simulink model "Plant_4"  (R2024b)
settings: Solver=VariableStepAuto  StartTime=0.0  StopTime=2  RelTol=1e-3
undefined symbols (not defined in the file or in its folder): g, I1, I2, L1, L2, lc1, lc2, m1, m2
libraries: slpidlib x2, simulink x2
settings Model: Creator=Sez26  LastModifiedBy=Sez26

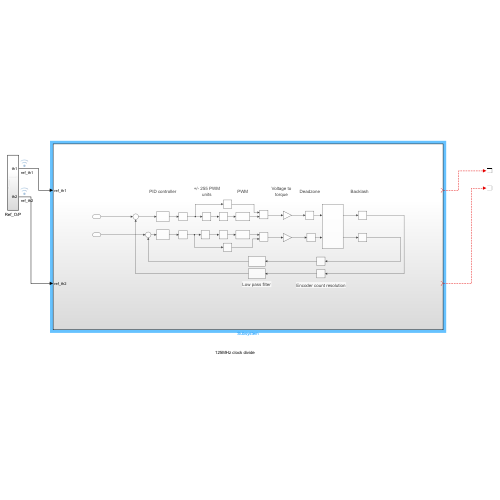
[thumbnail: Simulink's stored preview of the top-level diagram]
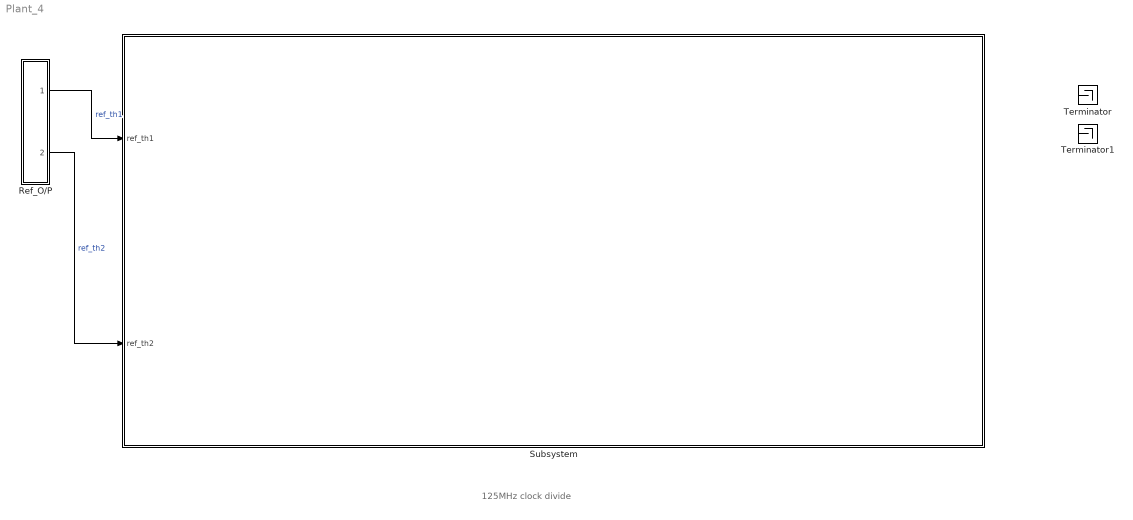
== system Plant_4 ==
  note: 125MHz clock divide
  Ref_O/P : Subsystem
  Subsystem : Subsystem
  Terminator : Terminator
  Terminator1 : Terminator
  wires:
  Ref_O/P/1(th1) -> Subsystem/1(ref_th1)  "ref_th1"
  Ref_O/P/2(th2) -> Subsystem/2(ref_th2)  "ref_th2"
  ? -> Terminator/1
  ? -> Terminator1/1

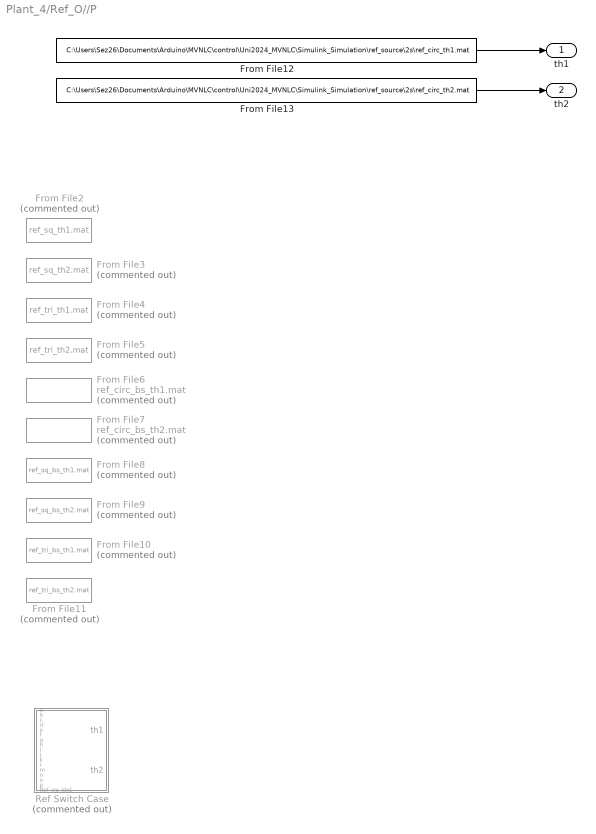
== system Plant_4/Ref_O//P ==
  From File10 : FromFile  Commented=on  FileName=ref_tri_bs_th1.mat  SampleTime=0
  From File11 : FromFile  Commented=on  FileName=ref_tri_bs_th2.mat  SampleTime=0
  From File12 : FromFile  FileName=C:\Users\Sez26\Documents\Arduino\MVNLC\control\Uni2024_MVNLC\Simulink_Simulation\ref_source\2s\ref_circ_th1.mat  SampleTime=0
  From File13 : FromFile  FileName=C:\Users\Sez26\Documents\Arduino\MVNLC\control\Uni2024_MVNLC\Simulink_Simulation\ref_source\2s\ref_circ_th2.mat  SampleTime=0
  From File2 : FromFile  Commented=on  FileName=ref_sq_th1.mat  SampleTime=0
  From File3 : FromFile  Commented=on  FileName=ref_sq_th2.mat  SampleTime=0
  From File4 : FromFile  Commented=on  FileName=ref_tri_th1.mat  SampleTime=0
  From File5 : FromFile  Commented=on  FileName=ref_tri_th2.mat  SampleTime=0
  From File6 : FromFile  Commented=on  FileName=ref_circ_bs_th1.mat  SampleTime=0
  From File7 : FromFile  Commented=on  FileName=ref_circ_bs_th2.mat  SampleTime=0
  From File8 : FromFile  Commented=on  FileName=ref_sq_bs_th1.mat  SampleTime=0
  From File9 : FromFile  Commented=on  FileName=ref_sq_bs_th2.mat  SampleTime=0
  Ref Switch Case : MATLAB Function  Commented=on  TreatAsAtomicUnit=on
  th1 : Outport
  th2 : Outport  Port=2
  wires:
  From File12/1 -> th1/1
  From File13/1 -> th2/1

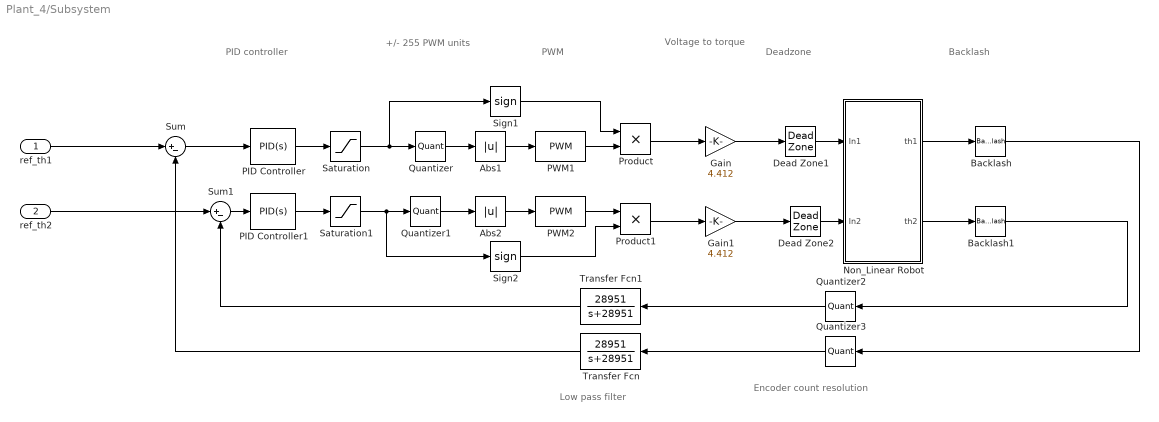
== system Plant_4/Subsystem ==
  note: PID controller
  note: +/- 255 PWM
      | units
  note: PWM
  note: Voltage to
      | torque
  note: Deadzone
  note: Low pass filter
  note: Encoder count resolution
  note: Backlash
  ref_th1 : Inport
  ref_th2 : Inport  Port=2
  Abs1 : Abs  SaturateOnIntegerOverflow=off
  Abs2 : Abs  SaturateOnIntegerOverflow=off
  Backlash : Backlash
  Backlash1 : Backlash
  Dead Zone1 : DeadZone  LowerValue=-(2.1/12)*4.4129925  UpperValue=(2.1/12)*4.4129925
  Dead Zone2 : DeadZone  LowerValue=-(2.1/12)*4.4129925  UpperValue=(2.1/12)*4.4129925
  Gain : Gain  Gain=4.412
  Gain1 : Gain  Gain=4.412
  Non_Linear Robot : Subsystem
  PID Controller : slpidlib/PID Controller  Controller=PID  Form=Parallel  TimeDomain=Continuous-time  UseExternalTs=off  SampleTime=-1  IntegratorMethod=Forward Euler  FilterMethod=Forward Euler  ControllerParametersSource=internal  P=300  I=0.1  UseKiTs=off  D=10  UseExternalDerivativeSource=off  N=100  UseFilter=on  TunerSelectOption=Transfer Function Based (PID Tuner App)  InitialConditionSource=internal  InitialConditionForIntegrator=0  InitialConditionForFilter=0  DifferentiatorICPrevScaledInput=0  ExternalReset=none  TrackingMode=off  Kt=1  LimitOutput=off  SatLimitsSource=internal  UpperSaturationLimit=1  LowerSaturationLimit=-1  LinearizeAsGain=on  AntiWindupMode=none  Kb=1  LimitIntegrator=off  UpperIntegratorSaturationLimit=inf  LowerIntegratorSaturationLimit=-inf  POutMin=[]  POutMax=[]  IOutMin=[]  IOutMax=[]  DOutMin=[]  DOutMax=[]  NOutMin=[]  NOutMax=[]  SumOutMin=[]  SumOutMax=[]  SaturationOutMin=[]  SaturationOutMax=[]  PParamMin=[]  PParamMax=[]  IParamMin=[]  IParamMax=[]  DParamMin=[]  DParamMax=[]  NParamMin=[]  NParamMax=[]  KbParamMin=[]  KbParamMax=[]  KtParamMin=[]  KtParamMax=[]  KbOutMin=[]  KbOutMax=[]  KtOutMin=[]  KtOutMax=[]  IntegratorOutMin=[]  IntegratorOutMax=[]  FilterOutMin=[]  FilterOutMax=[]  SumI1OutMin=[]  SumI1OutMax=[]  SumI2OutMin=[]  SumI2OutMax=[]  SumI3OutMin=[]  SumI3OutMax=[]  SumI4OutMin=[]  SumI4OutMax=[]  SumDOutMin=[]  SumDOutMax=[]  DifferentiatorOutMin=[]  DifferentiatorOutMax=[]  FilterDiffOutCoefMin=[]  FilterDiffOutCoefMax=[]  ReciprocalOutMin=[]  ReciprocalOutMax=[]  SumDenOutMin=[]  SumDenOutMax=[]  SumNumOutMin=[]  SumNumOutMax=[]  DivideOutMin=[]  DivideOutMax=[]  UdiffTsProdOutMin=[]  UdiffTsProdOutMax=[]  NTsProdOutMin=[]  NTsProdOutMax=[]  UintegralTsProdOutMin=[]  UintegralTsProdOutMax=[]  UngainTsProdOutMin=[]  UngainTsProdOutMax=[]  ClampingZeroOutDataTypeStr=Inherit: Inherit via back propagation  ClampingZeroOutMin=[]  ClampingZeroOutMax=[]  FilterDenConstantOutDataTypeStr=Inherit: Inherit via back propagation  FilterDenConstantOutMin=[]  FilterDenConstantOutMax=[]  PCopyOutDataTypeStr=Inherit: Inherit via back propagation  PCopyOutMin=[]  PCopyOutMax=[]  NCopyOutDataTypeStr=Inherit: Inherit via back propagation  NCopyOutMin=[]  NCopyOutMax=[]  IntegratorContinuousStateAttributes=''  IntegratorStateMustResolveToSignalObject=off  IntegratorRTWStateStorageClass=Auto  FilterContinuousStateAttributes=''  FilterStateMustResolveToSignalObject=off  FilterRTWStateStorageClass=Auto  ParallelPVariant=InternalParameters  IdealPVariant=Disabled  IVariant=InternalParameters  DVariant=InternalParameters  IntegratorVariant=Continuous  SatVariant=Disabled  AWVariant=Passthrough  PCopyVariant=Disabled  TRVariant=Disabled  FdbkBlocksVariant=Forward  IdealPFdbkVariant=Disabled  SatFdbkVariant=Disabled  DerivativeFilterVariant=ContFilter  NVariant=InternalParameters  NCopyVariant=Disabled  FilterICVariant=InternalICsFilter  IntegratorICVariant=InternalICs  ExternalResetVariant=Disabled  TRSumVariant=Passthrough  SumFdbkVariant=Disabled  SumVariant=Sum_PID  TsampFilterVariant=InternalTs  TsampNgainVariant=Passthrough  TsampIntegralVariant=Disabled_SignalSpec  ExternalSaturationOutDataTypeStr=Inherit: Same as second input  DerivativeSourceVariant=ErrorSignal  PreIntVariant=InternalPreInt
  PID Controller1 : slpidlib/PID Controller  Controller=PID  Form=Parallel  TimeDomain=Continuous-time  UseExternalTs=off  SampleTime=-1  IntegratorMethod=Forward Euler  FilterMethod=Forward Euler  ControllerParametersSource=internal  P=300  I=0.1  UseKiTs=off  D=10  UseExternalDerivativeSource=off  N=100  UseFilter=on  TunerSelectOption=Transfer Function Based (PID Tuner App)  InitialConditionSource=internal  InitialConditionForIntegrator=0  InitialConditionForFilter=0  DifferentiatorICPrevScaledInput=0  ExternalReset=none  TrackingMode=off  Kt=1  LimitOutput=off  SatLimitsSource=internal  UpperSaturationLimit=1  LowerSaturationLimit=-1  LinearizeAsGain=on  AntiWindupMode=none  Kb=1  LimitIntegrator=off  UpperIntegratorSaturationLimit=inf  LowerIntegratorSaturationLimit=-inf  POutMin=[]  POutMax=[]  IOutMin=[]  IOutMax=[]  DOutMin=[]  DOutMax=[]  NOutMin=[]  NOutMax=[]  SumOutMin=[]  SumOutMax=[]  SaturationOutMin=[]  SaturationOutMax=[]  PParamMin=[]  PParamMax=[]  IParamMin=[]  IParamMax=[]  DParamMin=[]  DParamMax=[]  NParamMin=[]  NParamMax=[]  KbParamMin=[]  KbParamMax=[]  KtParamMin=[]  KtParamMax=[]  KbOutMin=[]  KbOutMax=[]  KtOutMin=[]  KtOutMax=[]  IntegratorOutMin=[]  IntegratorOutMax=[]  FilterOutMin=[]  FilterOutMax=[]  SumI1OutMin=[]  SumI1OutMax=[]  SumI2OutMin=[]  SumI2OutMax=[]  SumI3OutMin=[]  SumI3OutMax=[]  SumI4OutMin=[]  SumI4OutMax=[]  SumDOutMin=[]  SumDOutMax=[]  DifferentiatorOutMin=[]  DifferentiatorOutMax=[]  FilterDiffOutCoefMin=[]  FilterDiffOutCoefMax=[]  ReciprocalOutMin=[]  ReciprocalOutMax=[]  SumDenOutMin=[]  SumDenOutMax=[]  SumNumOutMin=[]  SumNumOutMax=[]  DivideOutMin=[]  DivideOutMax=[]  UdiffTsProdOutMin=[]  UdiffTsProdOutMax=[]  NTsProdOutMin=[]  NTsProdOutMax=[]  UintegralTsProdOutMin=[]  UintegralTsProdOutMax=[]  UngainTsProdOutMin=[]  UngainTsProdOutMax=[]  ClampingZeroOutDataTypeStr=Inherit: Inherit via back propagation  ClampingZeroOutMin=[]  ClampingZeroOutMax=[]  FilterDenConstantOutDataTypeStr=Inherit: Inherit via back propagation  FilterDenConstantOutMin=[]  FilterDenConstantOutMax=[]  PCopyOutDataTypeStr=Inherit: Inherit via back propagation  PCopyOutMin=[]  PCopyOutMax=[]  NCopyOutDataTypeStr=Inherit: Inherit via back propagation  NCopyOutMin=[]  NCopyOutMax=[]  IntegratorContinuousStateAttributes=''  IntegratorStateMustResolveToSignalObject=off  IntegratorRTWStateStorageClass=Auto  FilterContinuousStateAttributes=''  FilterStateMustResolveToSignalObject=off  FilterRTWStateStorageClass=Auto  ParallelPVariant=InternalParameters  IdealPVariant=Disabled  IVariant=InternalParameters  DVariant=InternalParameters  IntegratorVariant=Continuous  SatVariant=Disabled  AWVariant=Passthrough  PCopyVariant=Disabled  TRVariant=Disabled  FdbkBlocksVariant=Forward  IdealPFdbkVariant=Disabled  SatFdbkVariant=Disabled  DerivativeFilterVariant=ContFilter  NVariant=InternalParameters  NCopyVariant=Disabled  FilterICVariant=InternalICsFilter  IntegratorICVariant=InternalICs  ExternalResetVariant=Disabled  TRSumVariant=Passthrough  SumFdbkVariant=Disabled  SumVariant=Sum_PID  TsampFilterVariant=InternalTs  TsampNgainVariant=Passthrough  TsampIntegralVariant=Disabled_SignalSpec  ExternalSaturationOutDataTypeStr=Inherit: Same as second input  DerivativeSourceVariant=ErrorSignal  PreIntVariant=InternalPreInt
  PWM1 : simulink/Discontinuities/PWM  DisableCoverage=on  Period=0.01  InitialDelay=0  DisallowZeroDutyCycle=off  RunAtFixedTimeIntervals=off  SampleTime=0.1
  PWM2 : simulink/Discontinuities/PWM  DisableCoverage=on  Period=0.01  InitialDelay=0  DisallowZeroDutyCycle=off  RunAtFixedTimeIntervals=off  SampleTime=0.1
  Product : Product
  Product1 : Product
  Quantizer : Quantizer  QuantizationInterval=1/(2*255)
  Quantizer1 : Quantizer  QuantizationInterval=1/(2*255)
  Quantizer2 : Quantizer  QuantizationInterval=360/(131.25*16)
  Quantizer3 : Quantizer  QuantizationInterval=360/(131.25*16)
  Saturation : Saturate  UpperLimit=1  LowerLimit=-1
  Saturation1 : Saturate  UpperLimit=1  LowerLimit=-1
  Sign1 : Signum
  Sign2 : Signum
  Sum : Sum  Inputs=|+-
  Sum1 : Sum  Inputs=|+-
  Transfer Fcn : TransferFcn  Numerator=28951  Denominator=[1 28951]
  Transfer Fcn1 : TransferFcn  Numerator=28951  Denominator=[1 28951]
  wires:
  Dead Zone1/1 -> Non_Linear Robot/1(In1)
  Quantizer1/1 -> Abs2/1
  Saturation/1 -> Quantizer/1, Sign1/1
  Product/1 -> Gain/1
  Abs2/1 -> PWM2/1
  Sign1/1 -> Product/1
  Quantizer/1 -> Abs1/1
  Saturation1/1 -> Quantizer1/1, Sign2/1
  Gain/1 -> Dead Zone1/1
  Sum1/1 -> PID Controller1/1
  Quantizer3/1 -> Transfer Fcn/1
  Product1/1 -> Gain1/1
  Quantizer2/1 -> Transfer Fcn1/1
  PWM1/1 -> Product/2
  PID Controller/1 -> Saturation/1
  Gain1/1 -> Dead Zone2/1
  Abs1/1 -> PWM1/1
  PID Controller1/1 -> Saturation1/1
  ref_th1/1 -> Sum/1
  Dead Zone2/1 -> Non_Linear Robot/2(In2)
  Sum/1 -> PID Controller/1
  ref_th2/1 -> Sum1/1
  PWM2/1 -> Product1/1
  Sign2/1 -> Product1/2
  Non_Linear Robot/1(th1) -> Backlash/1
  Non_Linear Robot/2(th2) -> Backlash1/1
  Backlash/1 -> Quantizer3/1
  Backlash1/1 -> Quantizer2/1
  Transfer Fcn1/1 -> Sum1/2
  Transfer Fcn/1 -> Sum/2

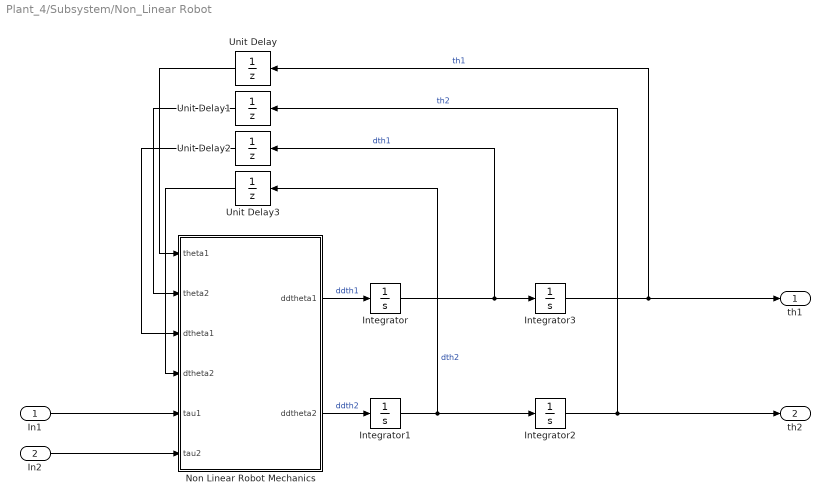
== system Plant_4/Subsystem/Non_Linear Robot ==
  In1 : Inport
  In2 : Inport  Port=2
  Integrator{,1..3} (4 alike) : Integrator
  Non Linear Robot Mechanics : MATLAB Function  TreatAsAtomicUnit=on
  Unit Delay{,1..3} (4 alike) : UnitDelay  SampleTime=-1  HasFrameUpgradeWarning=on
  th1 : Outport
  th2 : Outport  Port=2
  wires:
  Integrator1/1 -> Unit Delay3/1, Integrator2/1  "dth2"
  Integrator2/1 -> Unit Delay1/1, th2/1  "th2"
  Integrator3/1 -> Unit Delay/1, th1/1  "th1"
  Non Linear Robot Mechanics/1(ddtheta1) -> Integrator/1  "ddth1"
  In2/1 -> Non Linear Robot Mechanics/6(tau2)
  In1/1 -> Non Linear Robot Mechanics/5(tau1)
  Integrator/1 -> Unit Delay2/1, Integrator3/1  "dth1"
  Non Linear Robot Mechanics/2(ddtheta2) -> Integrator1/1  "ddth2"
  Unit Delay3/1 -> Non Linear Robot Mechanics/4(dtheta2)
  Unit Delay2/1 -> Non Linear Robot Mechanics/3(dtheta1)
  Unit Delay1/1 -> Non Linear Robot Mechanics/2(theta2)
  Unit Delay/1 -> Non Linear Robot Mechanics/1(theta1)

== matlab function Plant_4/Subsystem/Non_Linear Robot/Non Linear Robot Mechanics ==
  data: theta1 input; theta2 input; dtheta1 input; dtheta2 input; ddtheta1 output; tau1 input; tau2 input; m2 parameter; m1 parameter; L1 parameter; L2 parameter; I1 parameter; I2 parameter; g parameter; lc1 parameter; lc2 parameter; ddtheta2 output
function [ddtheta1, ddtheta2]= Robot_SS(theta1, theta2, dtheta1, dtheta2, tau1, tau2, m2, m1, L1, L2, I1, I2, g, lc1, lc2)
    % Mass matrix M(theta)
    M11 = m1 * lc1^2 + m2 * (L1^2 + lc2^2 + 2 * L1 * lc2 * cos(theta2)) + I1 + I2;
    M12 = m2 * (lc2^2 + L1 * lc2 * cos(theta2)) + I2;
    M21 = M12;
    M22 = m2 * lc2^2 + I2;
    M = [M11, M12; M21, M22];
    
    % Coriolis matrix C(theta, omega)
    C11 = -m2 * L1 * lc2 * sin(theta2) * dtheta2;
    C12 = -m2 * L1 * lc2 * sin(theta2) * (dtheta1 + dtheta2);
    C21 = m2 * L1 * lc2 * sin(theta2) * dtheta1;
    C22 = 0;
    C = [C11, C12; C21, C22];
    
    % Gravity vector G(theta)
    G1 = (m1 * lc1 + m2 * L1) * g * cos(theta1) + m2 * lc2 * g * cos(theta1 + theta2);
    G2 = m2 * lc2 * g * cos(theta1 + theta2);
    G = [G1; G2];
    
    % Solve for angular accelerations: M * ddtheta = tau - C * dtheta - G
    tau = [tau1; tau2];
    theta_dot = [dtheta1; dtheta2];
    ddtheta = M\(tau - C * theta_dot - G);
    ddtheta1 = ddtheta(1);
    ddtheta2 = ddtheta(2);

    % calculate new
    % % State-space matrices
    % A = zeros(4, 4);
    % A(1, 3) = 1;
    % A(2, 4) = 1;
    % A(3:4, 3:4) = -M \ C;
    % 
    % B = zeros(4, 2);
    % B(3:4, :) = M \ eye(2);
end

== matlab function Plant_4/Ref_O//P/Ref Switch Case ==
  data: Ref_sig_idx parameter; a input; b input; c input; d input; e input; f input; g input; h input; i input; j input; k input; l input; m input; n input; o input; p input; Ref_sig_idx1 input; th1 output; th2 output
function [th1, th2] = ref_switch(Ref_sig_idx, a, b, c, d, e, f, g, h, i, j, k, l, m, n, o, p, Ref_sig_idx1)
    if Ref_sig_idx == 0
        % circ base
        th1 = a;
        th2 = b;
    elseif Ref_sig_idx == 1
        % sq base
        th1 = c;
        th2 = d;
    elseif Ref_sig_idx == 2
        % tri base
        th1 = e;
        th2 = f;
    end
    if Ref_sig_idx == 3
        % circ b spline
        th1 = g;
        th2 = h;
    elseif Ref_sig_idx == 4
        % sq b spline
        th1 = i;
        th2 = j;
    elseif Ref_sig_idx == 5
        % tri b spline
        th1 = k;
        th2 = l;
    end
    if Ref_sig_idx == 6
        % sq corner sf
        th1 = m;
        th2 = n;
    elseif Ref_sig_idx == 7
        % tri corner sf
        th1 = o;
        th2 = p;
    else
        % invalid reference choice
        disp('Error invalid reference choice')
        th1 = 0;
        th2 = 0;
    end
